simulink model "SPGF_FSK_0000_R2021b"  (R2021b)
settings: Solver=ode4  StartTime=0.0  StopTime=1.4  FixedStep=50e-6/50  RelTol=1e-3  EnableMultiTasking=on
undefined symbols (not defined in the file): D11, Delta
libraries: spsSeriesRLCBranchLib x1645, spsGroundLib x359, spsCurrentMeasurementLib x145, spsIdealSwitchLib x144, spsStairGeneratorLib x135, spsUniversalBridgeLib x76, spsThreePhaseSeriesRLCLoadLib x57, spsSequenceAnalyzerLib x31, simulink x24, spsThreePhaseParallelRLCLoadLib x20, spsThreePhaseTransformerTwoWindingsLib x20, spsDistributedParametersLineLib x19
(part 12 of 36)

== system SPGF_FSK_0000_R2021b/W11/DPL ==
  Ccs2/1 : spsSeriesRLCBranchLib/Series RLC Branch  LConnTagsString=__new0  RConnTagsString=__new0  BranchType=R  Resistance=-Rg_matrix(3,4)*2  Inductance=1e-3  SetiL0=off  InitialCurrent=0  Capacitance=Rg_matrix(3,4)*2  Setx0=off  InitialVoltage=0  Measurements=None
  Ccs2/3 : spsSeriesRLCBranchLib/Series RLC Branch  LConnTagsString=__new0  RConnTagsString=__new0  BranchType=R  Resistance=-Rg_matrix(3,4)*2  Inductance=1e-3  SetiL0=off  InitialCurrent=0  Capacitance=Rg_matrix(3,4)*2  Setx0=off  InitialVoltage=0  Measurements=None
  Ccs3/1 : spsSeriesRLCBranchLib/Series RLC Branch  LConnTagsString=__new0  RConnTagsString=__new0  BranchType=R  Resistance=-Rg_matrix(5,6)*2  Inductance=1e-3  SetiL0=off  InitialCurrent=0  Capacitance=-C_matrix(5,6)/2  Setx0=off  InitialVoltage=0  Measurements=None
  Ccs3/3 : spsSeriesRLCBranchLib/Series RLC Branch  LConnTagsString=__new0  RConnTagsString=__new0  BranchType=R  Resistance=-Rg_matrix(5,6)*2  Inductance=1e-3  SetiL0=off  InitialCurrent=0  Capacitance=-C_matrix(5,6)/2  Setx0=off  InitialVoltage=0  Measurements=None
  DPL : spsDistributedParametersLineLib/Distributed Parameters Line  Phases=6  Length=LineLength  Frequency=Frequency  Resistance=R_matrix  Inductance=L_matrix  Capacitance=C_matrix  x1=[-0.0001055 -1.78412619667985 4844.51130994743 0 0 0 -9280.60987849936;-0.000105 -1.78462942618335 4845.96807552508 0 0 0 -9279.84399978977;-0.0001045 -1.78513261165289 4847.42472153325 0 0 0 -9279.07789210921;-0.000104 -1.78563575307605 4848.88124793602 0 0 0 -9278.31155547658;-0.0001035 -1.78613885044041 4850.33765469743 0 0 0 -9277.54498991079;-0.000103 -1.78664190373356 4851.79394178156 0 0 0 -9276.77819543075;-0.0001025 -1.78714491294309 4853.25010915248 0 0 0 -9276.01117205539;-0.000102 -1.78764787805659 4854.70615677424 0 0 0 -9275.24391980362;-0.0001015 -1.78815079906164 4856.16208461094 0 0 0 -9274.47643869439;-0.000101 -1.78865367594584 4857.61789262663 0 0 0 -9273.70872874662;-0.0001005 -1.78915650869679 4859.07358078542 0 0 0 -9272.94078997926;-0.0001 -1.78965929730206 4860.52914905136 0 0 0 -9272.17262241126;-9.95e-05 -1.79016204174926 4861.98459738856 0 0 0 -9271.40422606157;-9.9e-05 -1.79066474202598 4863.43992576109 0 0 0 -9270.63560094915;-9.85e-05 -1.79116739811982 4864.89513413306 0 0 0 -9269.86674709296;-9.8e-05 -1.79167001001838 4866.35022246855 0 0 0 -9269.09766451198;-9.75e-05 -1.79217257770925 4867.80519073166 0 0 0 -9268.32835322519;-9.7e-05 -1.79267510118004 4869.26003888649 0 0 0 -9267.55881325156;-9.65e-05 -1.79317758041834 4870.71476689715 0 0 0 -9266.78904461008;-9.6e-05 -1.79368001541176 4872.16937472774 0 0 0 -9266.01904731975;-9.55e-05 -1.79418240614789 4873.62386234236 0 0 0 -9265.24882139956;-9.5e-05 -1.79468475261435 4875.07822970514 0 0 0 -9264.47836686852;-9.45e-05 -1.79518705479874 4876.53247678019 0 0 0 -9263.70768374564;-9.4e-05 -1.79568931268867 4877.98660353161 0 0 0 -9262.93677204993;-9.35e-05 -1.79619152627174 4879.44060992355 0 0 0 -9262.16563180043;-9.3e-05 -1.79669369553555 4880.89449592011 0 0 0 -9261.39426301614;-9.25e-05 -1.79719582046773 4882.34826148543 0 0 0 -9260.62266571611;-9.2e-05 -1.79769790105588 4883.80190658364 0 0 0 -9259.85083991938;-9.15e-05 -1.79819993728761 4885.25543117886 0 0 0 -9259.07878564499;-9.1e-05 -1.79870192915053 4886.70883523523 0 0 0 -9258.30650291198;-9.05e-05 -1.79920387663227 4888.1621187169 0 0 0 -9257.53399173942;-9e-05 -1.79970577972043 4889.61528158801 0 0 0 -9256.76125214637;-8.95e-05 -1.80020763840262 4891.06832381269 0 0 0 -9255.98828415188;-8.9e-05 -1.80070945266648 4892.5212453551 0 0 0 -9255.21508777504;-8.85e-05 -1.80121122249961 4893.97404617938 0 0 0 -9254.44166303492;-8.8e-05 -1.80171294788964 4895.4267262497 0 0 0 -9253.6680099506;-8.75e-05 -1.80221462882418 4896.87928553021 0 0 0 -9252.89412854118;-8.7e-05 -1.80271626529085 4898.33172398506 0 0 0 -9252.12001882575;-8.65e-05 -1.80321785727729 4899.78404157842 0 0 0 -9251.34568082341;-8.6e-05 -1.80371940477111 4901.23623827445 0 0 0 -9250.57111455326;-8.55e-05 -1.80422090775993 4902.68831403733 0 0 0 -9249.79632003442;-8.5e-05 -1.80472236623139 4904.14026883123 0 0 0 -9249.02129728601;-8.45e-05 -1.80522378017311 4905.59210262031 0 0 0 -9248.24604632714;-8.4e-05 -1.80572514957272 4907.04381536876 0 0 0 -9247.47056717695;-8.35e-05 -1.80622647441785 4908.49540704076 0 0 0 -9246.69485985456;-8.3e-05 -1.80672775469612 4909.94687760048 0 0 0 -9245.91892437913;-8.25e-05 -1.80722899039518 4911.39822701213 0 0 0 -9245.14276076979;-8.2e-05 -1.80773018150264 4912.84945523988 0 0 0 -9244.3663690457;-8.15e-05 -1.80823132800616 4914.30056224793 0 0 0 -9243.58974922601;-8.1e-05 -1.80873242989335 4915.75154800047 0 0 0 -9242.81290132989;-8.05e-05 -1.80923348715186 4917.20241246171 0 0 0 -9242.0358253765;-8e-05 -1.80973449976932 4918.65315559584 0 0 0 -9241.25852138502;-7.95e-05 -1.81023546773337 4920.10377736707 0 0 0 -9240.48098937462;-7.9e-05 -1.81073639103166 4921.5542777396 0 0 0 -9239.70322936449;-7.85e-05 -1.81123726965181 4923.00465667765 0 0 0 -9238.92524137383;-7.8e-05 -1.81173810358148 4924.45491414543 0 0 0 -9238.14702542182;-7.75e-05 -1.8122388928083 4925.90505010715 0 0 0 -9237.36858152767;-7.7e-05 -1.81273963731991 4927.35506452704 0 0 0 -9236.58990971059;-7.65e-05 -1.81324033710397 ...(+12181 chars)]  x2=[-0.0001055 -1.77906835575681 4945.74076916884 0 0 0 -9459.89906055918;-0.000105 -1.7795989916804 4947.22756988038 0 0 0 -9459.12257831348;-0.0001045 -1.78012958369414 4948.71424852397 0 0 0 -9458.34586267329;-0.000104 -1.78066013178495 4950.20080506292 0 0 0 -9457.56891365777;-0.0001035 -1.78119063593973 4951.68723946057 0 0 0 -9456.79173128609;-0.000103 -1.78172109614539 4953.17355168024 0 0 0 -9456.01431557743;-0.0001025 -1.78225151238884 4954.65974168524 0 0 0 -9455.23666655097;-0.000102 -1.782781884657 4956.14580943892 0 0 0 -9454.4587842259;-0.0001015 -1.78331221293679 4957.6317549046 0 0 0 -9453.68066862141;-0.000101 -1.7838424972151 4959.11757804562 0 0 0 -9452.90231975669;-0.0001005 -1.78437273747887 4960.60327882532 0 0 0 -9452.12373765096;-0.0001 -1.78490293371501 4962.08885720704 0 0 0 -9451.34492232343;-9.95e-05 -1.78543308591043 4963.57431315412 0 0 0 -9450.56587379331;-9.9e-05 -1.78596319405205 4965.05964662992 0 0 0 -9449.78659207982;-9.85e-05 -1.7864932581268 4966.54485759778 0 0 0 -9449.00707720219;-9.8e-05 -1.7870232781216 4968.02994602106 0 0 0 -9448.22732917966;-9.75e-05 -1.78755325402336 4969.51491186311 0 0 0 -9447.44734803147;-9.7e-05 -1.78808318581901 4970.9997550873 0 0 0 -9446.66713377685;-9.65e-05 -1.78861307349548 4972.48447565699 0 0 0 -9445.88668643507;-9.6e-05 -1.7891429170397 4973.96907353554 0 0 0 -9445.10600602538;-9.55e-05 -1.78967271643858 4975.45354868632 0 0 0 -9444.32509256703;-9.5e-05 -1.79020247167905 4976.93790107271 0 0 0 -9443.54394607931;-9.45e-05 -1.79073218274805 4978.42213065807 0 0 0 -9442.76256658148;-9.4e-05 -1.79126184963251 4979.9062374058 0 0 0 -9441.98095409282;-9.35e-05 -1.79179147231935 4981.39022127926 0 0 0 -9441.19910863263;-9.3e-05 -1.79232105079551 4982.87408224185 0 0 0 -9440.41703022018;-9.25e-05 -1.79285058504792 4984.35782025695 0 0 0 -9439.63471887477;-9.2e-05 -1.79338007506351 4985.84143528794 0 0 0 -9438.85217461572;-9.15e-05 -1.79390952082923 4987.32492729823 0 0 0 -9438.06939746233;-9.1e-05 -1.794438922332 4988.80829625122 0 0 0 -9437.28638743391;-9.05e-05 -1.79496827955876 4990.29154211029 0 0 0 -9436.50314454978;-9e-05 -1.79549759249646 4991.77466483885 0 0 0 -9435.71966882926;-8.95e-05 -1.79602686113203 4993.25766440031 0 0 0 -9434.9359602917;-8.9e-05 -1.79655608545242 4994.74054075808 0 0 0 -9434.15201895643;-8.85e-05 -1.79708526544456 4996.22329387556 0 0 0 -9433.36784484278;-8.8e-05 -1.7976144010954 4997.70592371617 0 0 0 -9432.58343797011;-8.75e-05 -1.79814349239188 4999.18843024334 0 0 0 -9431.79879835778;-8.7e-05 -1.79867253932095 5000.67081342047 0 0 0 -9431.01392602514;-8.65e-05 -1.79920154186955 5002.153073211 0 0 0 -9430.22882099156;-8.6e-05 -1.79973050002464 5003.63520957835 0 0 0 -9429.4434832764;-8.55e-05 -1.80025941377315 5005.11722248594 0 0 0 -9428.65791289906;-8.5e-05 -1.80078828310204 5006.59911189723 0 0 0 -9427.87210987891;-8.45e-05 -1.80131710799827 5008.08087777562 0 0 0 -9427.08607423534;-8.4e-05 -1.80184588844877 5009.56252008458 0 0 0 -9426.29980598774;-8.35e-05 -1.80237462444052 5011.04403878754 0 0 0 -9425.51330515552;-8.3e-05 -1.80290331596045 5012.52543384794 0 0 0 -9424.72657175808;-8.25e-05 -1.80343196299552 5014.00670522923 0 0 0 -9423.93960581483;-8.2e-05 -1.80396056553269 5015.48785289487 0 0 0 -9423.1524073452;-8.15e-05 -1.80448912355892 5016.9688768083 0 0 0 -9422.3649763686;-8.1e-05 -1.80501763706117 5018.44977693299 0 0 0 -9421.57731290446;-8.05e-05 -1.80554610602639 5019.9305532324 0 0 0 -9420.78941697222;-8e-05 -1.80607453044155 5021.41120566998 0 0 0 -9420.00128859132;-7.95e-05 -1.8066029102936 5022.89173420921 0 0 0 -9419.21292778121;-7.9e-05 -1.80713124556952 5024.37213881355 0 0 0 -9418.42433456133;-7.85e-05 -1.80765953625626 5025.85241944648 0 0 0 -9417.63550895114;-7.8e-05 -1.80818778234078 5027.33257607148 0 0 0 -9416.84645097012;-7.75e-05 -1.80871598381007 5028.81260865201 0 0 0 -9416.05716063772;-7.7e-05 -1.80924414065107 5030.29251715156 0 0 0 -9415.26763797342;-7.65e-05 -1.80977225285076 ...(+12156 chars)]  x3=[-0.0001055 0.0207090066909794 -36.7832656385474 0 0 0 -561.751834737637;-0.000105 0.0207044314271113 -36.6997989422163 0 0 0 -561.75382588602;-0.0001045 0.0206998556523819 -36.616331340354 0 0 0 -561.755803173683;-0.000104 0.0206952793669039 -36.5328628350199 0 0 0 -561.757766600577;-0.0001035 0.0206907025707905 -36.4493934282735 0 0 0 -561.759716166653;-0.000103 0.0206861252641544 -36.3659231221744 0 0 0 -561.761651871865;-0.0001025 0.0206815474471086 -36.2824519187821 0 0 0 -561.763573716163;-0.000102 0.0206769691197661 -36.1989798201562 0 0 0 -561.7654816995;-0.0001015 0.0206723902822399 -36.1155068283563 0 0 0 -561.76737582183;-0.000101 0.0206678109346428 -36.0320329454419 0 0 0 -561.769256083106;-0.0001005 0.020663231077088 -35.9485581734728 0 0 0 -561.771122483281;-0.0001 0.0206586507096883 -35.8650825145086 0 0 0 -561.772975022309;-9.95e-05 0.0206540698325569 -35.7816059706089 0 0 0 -561.774813700144;-9.9e-05 0.0206494884458068 -35.6981285438335 0 0 0 -561.776638516741;-9.85e-05 0.0206449065495509 -35.614650236242 0 0 0 -561.778449472056;-9.8e-05 0.0206403241439024 -35.5311710498943 0 0 0 -561.780246566043;-9.75e-05 0.0206357412289744 -35.4476909868501 0 0 0 -561.782029798658;-9.7e-05 0.0206311578048798 -35.3642100491692 0 0 0 -561.783799169857;-9.65e-05 0.0206265738717318 -35.2807282389114 0 0 0 -561.785554679596;-9.6e-05 0.0206219894296434 -35.1972455581365 0 0 0 -561.787296327833;-9.55e-05 0.0206174044787279 -35.1137620089044 0 0 0 -561.789024114524;-9.5e-05 0.0206128190190984 -35.0302775932749 0 0 0 -561.790738039626;-9.45e-05 0.0206082330508679 -34.946792313308 0 0 0 -561.792438103097;-9.4e-05 0.0206036465741496 -34.8633061710635 0 0 0 -561.794124304895;-9.35e-05 0.0205990595890567 -34.7798191686015 0 0 0 -561.795796644979;-9.3e-05 0.0205944720957025 -34.6963313079818 0 0 0 -561.797455123308;-9.25e-05 0.0205898840941999 -34.6128425912644 0 0 0 -561.79909973984;-9.2e-05 0.0205852955846624 -34.5293530205094 0 0 0 -561.800730494535;-9.15e-05 0.0205807065672031 -34.4458625977768 0 0 0 -561.802347387352;-9.1e-05 0.0205761170419351 -34.3623713251266 0 0 0 -561.803950418252;-9.05e-05 0.0205715270089719 -34.2788792046188 0 0 0 -561.805539587195;-9e-05 0.0205669364684265 -34.1953862383136 0 0 0 -561.807114894143;-8.95e-05 0.0205623454204124 -34.111892428271 0 0 0 -561.808676339055;-8.9e-05 0.0205577538650427 -34.0283977765513 0 0 0 -561.810223921894;-8.85e-05 0.0205531618024307 -33.9449022852145 0 0 0 -561.811757642621;-8.8e-05 0.0205485692326898 -33.8614059563208 0 0 0 -561.813277501199;-8.75e-05 0.0205439761559333 -33.7779087919304 0 0 0 -561.81478349759;-8.7e-05 0.0205393825722745 -33.6944107941035 0 0 0 -561.816275631757;-8.65e-05 0.0205347884818268 -33.6109119649004 0 0 0 -561.817753903662;-8.6e-05 0.0205301938847034 -33.5274123063812 0 0 0 -561.819218313271;-8.55e-05 0.0205255987810179 -33.4439118206063 0 0 0 -561.820668860546;-8.5e-05 0.0205210031708834 -33.360410509636 0 0 0 -561.822105545451;-8.45e-05 0.0205164070544135 -33.2769083755305 0 0 0 -561.823528367952;-8.4e-05 0.0205118104317216 -33.1934054203502 0 0 0 -561.824937328013;-8.35e-05 0.020507213302921 -33.1099016461555 0 0 0 -561.826332425599;-8.3e-05 0.0205026156681253 -33.0263970550067 0 0 0 -561.827713660676;-8.25e-05 0.0204980175274477 -32.9428916489642 0 0 0 -561.82908103321;-8.2e-05 0.0204934188810019 -32.8593854300884 0 0 0 -561.830434543167;-8.15e-05 0.0204888197289012 -32.7758784004398 0 0 0 -561.831774190514;-8.1e-05 0.0204842200712592 -32.6923705620789 0 0 0 -561.833099975217;-8.05e-05 0.0204796199081892 -32.608861917066 0 0 0 -561.834411897245;-8e-05 0.0204750192398049 -32.5253524674617 0 0 0 -561.835709956563;-7.95e-05 0.0204704180662198 -32.4418422153265 0 0 0 -561.836994153142;-7.9e-05 0.0204658163875474 -32.3583311627209 0 0 0 -561.838264486948;-7.85e-05 0.0204612142039011 -32.2748193117055 0 0 0 -561.839520957951;-7.8e-05 0.0204566115153947 -32.1913066643409 0 0 0 -561.840763566119;-7.75e-05 0.0204520083221416 -32.1077932226876 0 0 0 ...(+12583 chars)]  x4=[-0.0001055 -0.04304225965487 184.459272299607 0 0 0 227.528775566243;-0.000105 -0.0430444284629222 184.420510607988 0 0 0 227.558114219598;-0.0001045 -0.0430465962088957 184.381744365975 0 0 0 227.587447258182;-0.000104 -0.043048762892737 184.342973574525 0 0 0 227.61677468127;-0.0001035 -0.0430509285143927 184.304198234594 0 0 0 227.64609648814;-0.000103 -0.0430530930738093 184.26541834714 0 0 0 227.675412678067;-0.0001025 -0.0430552565709334 184.226633913118 0 0 0 227.704723250329;-0.000102 -0.0430574190057116 184.187844933487 0 0 0 227.734028204201;-0.0001015 -0.0430595803780906 184.149051409203 0 0 0 227.763327538962;-0.000101 -0.043061740688017 184.110253341223 0 0 0 227.792621253888;-0.0001005 -0.0430638999354376 184.071450730505 0 0 0 227.821909348257;-0.0001 -0.0430660581202991 184.032643578005 0 0 0 227.851191821345;-9.95e-05 -0.0430682152425481 183.993831884682 0 0 0 227.88046867243;-9.9e-05 -0.0430703713021315 183.955015651494 0 0 0 227.90973990079;-9.85e-05 -0.0430725262989961 183.916194879397 0 0 0 227.939005505703;-9.8e-05 -0.0430746802330888 183.87736956935 0 0 0 227.968265486446;-9.75e-05 -0.0430768331043563 183.838539722311 0 0 0 227.997519842298;-9.7e-05 -0.0430789849127455 183.799705339238 0 0 0 228.026768572537;-9.65e-05 -0.0430811356582034 183.760866421089 0 0 0 228.05601167644;-9.6e-05 -0.0430832853406769 183.722022968822 0 0 0 228.085249153287;-9.55e-05 -0.043085433960113 183.683174983396 0 0 0 228.114481002356;-9.5e-05 -0.0430875815164585 183.644322465769 0 0 0 228.143707222926;-9.45e-05 -0.0430897280096606 183.6054654169 0 0 0 228.172927814275;-9.4e-05 -0.0430918734396663 183.566603837748 0 0 0 228.202142775683;-9.35e-05 -0.0430940178064227 183.527737729272 0 0 0 228.231352106429;-9.3e-05 -0.0430961611098767 183.48886709243 0 0 0 228.260555805792;-9.25e-05 -0.0430983033499756 183.449991928182 0 0 0 228.289753873052;-9.2e-05 -0.0431004445266665 183.411112237487 0 0 0 228.318946307488;-9.15e-05 -0.0431025846398966 183.372228021304 0 0 0 228.348133108379;-9.1e-05 -0.043104723689613 183.333339280593 0 0 0 228.377314275007;-9.05e-05 -0.043106861675763 183.294446016312 0 0 0 228.40648980665;-9e-05 -0.0431089985982938 183.255548229423 0 0 0 228.435659702588;-8.95e-05 -0.0431111344571527 183.216645920884 0 0 0 228.464823962103;-8.9e-05 -0.0431132692522871 183.177739091656 0 0 0 228.493982584474;-8.85e-05 -0.0431154029836441 183.138827742698 0 0 0 228.523135568982;-8.8e-05 -0.0431175356511712 183.099911874971 0 0 0 228.552282914908;-8.75e-05 -0.0431196672548157 183.060991489434 0 0 0 228.581424621532;-8.7e-05 -0.0431217977945252 183.022066587049 0 0 0 228.610560688136;-8.65e-05 -0.0431239272702469 182.983137168775 0 0 0 228.639691114;-8.6e-05 -0.0431260556819283 182.944203235573 0 0 0 228.668815898406;-8.55e-05 -0.043128183029517 182.905264788404 0 0 0 228.697935040635;-8.5e-05 -0.0431303093129604 182.866321828228 0 0 0 228.727048539968;-8.45e-05 -0.0431324345322061 182.827374356007 0 0 0 228.756156395688;-8.4e-05 -0.0431345586872017 182.788422372701 0 0 0 228.785258607076;-8.35e-05 -0.0431366817778946 182.749465879272 0 0 0 228.814355173415;-8.3e-05 -0.0431388038042326 182.71050487668 0 0 0 228.843446093985;-8.25e-05 -0.0431409247661633 182.671539365887 0 0 0 228.872531368069;-8.2e-05 -0.0431430446636343 182.632569347855 0 0 0 228.90161099495;-8.15e-05 -0.0431451634965934 182.593594823545 0 0 0 228.930684973911;-8.1e-05 -0.0431472812649883 182.554615793918 0 0 0 228.959753304233;-8.05e-05 -0.0431493979687666 182.515632259937 0 0 0 228.988815985199;-8e-05 -0.0431515136078763 182.476644222563 0 0 0 229.017873016093;-7.95e-05 -0.043153628182265 182.437651682758 0 0 0 229.046924396198;-7.9e-05 -0.0431557416918806 182.398654641485 0 0 0 229.075970124796;-7.85e-05 -0.043157854136671 182.359653099705 0 0 0 229.105010201171;-7.8e-05 -0.043159965516584 182.320647058381 0 0 0 229.134044624607;-7.75e-05 -0.0431620758315675 182.281636518476 0 0 0 229.163073394387;-7.7e-05 -0.0431641850815695 182.242621480951 0 0 0 ...(+12359 chars)]  x5=0.000105022628283662  V1=ones(3,3)  V2=ones(3,3)  I1=ones(3,3)  I2=ones(3,3)  nHarmo=1  Measurements=None  Decoupling=off  VsMag0=0  VrMag0=0  VsAngle0=0  VrAngle0=0  IsMag0=0  IrMag0=0  IsAngle0=0  IrAngle0=0
  Ground{1..4} (4 alike) : spsGroundLib/Ground  LConnTagsString=a
  Rcs*1 : spsSeriesRLCBranchLib/Series RLC Branch  LConnTagsString=__new0  RConnTagsString=__new0  BranchType=R  Resistance=-Rg_matrix(1,2)*2  Inductance=1e-3  SetiL0=off  InitialCurrent=0  Capacitance=Rg_matrix(1,2)*2  Setx0=off  InitialVoltage=0  Measurements=None
  Rcs*2 : spsSeriesRLCBranchLib/Series RLC Branch  LConnTagsString=__new0  RConnTagsString=__new0  BranchType=R  Resistance=-Rg_matrix(1,2)*2  Inductance=1e-3  SetiL0=off  InitialCurrent=0  Capacitance=Rg_matrix(1,2)*2  Setx0=off  InitialVoltage=0  Measurements=None
  Rgsg1/1 : spsSeriesRLCBranchLib/Series RLC Branch  LConnTagsString=__new0  RConnTagsString=__new0  BranchType=R  Resistance=(Rg_matrix(4,4)+Rg_matrix(3,4))*2  Inductance=1e-3  SetiL0=off  InitialCurrent=0  Capacitance=Rg_matrix(1,2)*2  Setx0=off  InitialVoltage=0  Measurements=None
  Rgsg1/2 : spsSeriesRLCBranchLib/Series RLC Branch  LConnTagsString=__new0  RConnTagsString=__new0  BranchType=R  Resistance=(Rg_matrix(2,2)+Rg_matrix(1,2))*2  Inductance=1e-3  SetiL0=off  InitialCurrent=0  Capacitance=Rg_matrix(1,2)*2  Setx0=off  InitialVoltage=0  Measurements=None
  Rgsg1/3 : spsSeriesRLCBranchLib/Series RLC Branch  LConnTagsString=__new0  RConnTagsString=__new0  BranchType=R  Resistance=(Rg_matrix(4,4)+Rg_matrix(3,4))*2  Inductance=1e-3  SetiL0=off  InitialCurrent=0  Capacitance=Rg_matrix(1,2)*2  Setx0=off  InitialVoltage=0  Measurements=None
  Rgsg1/4 : spsSeriesRLCBranchLib/Series RLC Branch  LConnTagsString=__new0  RConnTagsString=__new0  BranchType=R  Resistance=(Rg_matrix(2,2)+Rg_matrix(1,2))*2  Inductance=1e-3  SetiL0=off  InitialCurrent=0  Capacitance=Rg_matrix(1,2)*2  Setx0=off  InitialVoltage=0  Measurements=None
  Rsg*1 : spsSeriesRLCBranchLib/Series RLC Branch  LConnTagsString=__new0  RConnTagsString=__new0  BranchType=R  Resistance=(Rg_matrix(6,6)+Rg_matrix(5,6))*2  Inductance=1e-3  SetiL0=off  InitialCurrent=0  Capacitance=Rg_matrix(1,2)*2  Setx0=off  InitialVoltage=0  Measurements=None
  Rsg*2 : spsSeriesRLCBranchLib/Series RLC Branch  LConnTagsString=__new0  RConnTagsString=__new0  BranchType=R  Resistance=(Rg_matrix(6,6)+Rg_matrix(5,6))*2  Inductance=1e-3  SetiL0=off  InitialCurrent=0  Capacitance=Rg_matrix(1,2)*2  Setx0=off  InitialVoltage=0  Measurements=None
  A : PMIOPort  Side=Left
  B : PMIOPort  Port=2  Side=Left
  C : PMIOPort  Port=3  Side=Left
  a : PMIOPort  Port=4  Side=Right
  b : PMIOPort  Port=5  Side=Right
  c : PMIOPort  Port=6  Side=Right
  connections:
  DPL/LConn2 -- Rgsg1/1/LConn1 -- Ccs2/3/LConn1 -- DPL/LConn4 -- Ccs3/3/LConn1 -- Rsg*2/LConn1 -- DPL/LConn6 -- Ground3/LConn1 -- Rgsg1/2/LConn1 -- Rcs*2/LConn1
  DPL/RConn5 -- c/RConn1 -- Ccs3/1/RConn1
  Ccs2/1/RConn1 -- b/RConn1 -- DPL/RConn3
  DPL/RConn1 -- a/RConn1 -- Rcs*1/RConn1
  DPL/RConn6 -- Ground4/LConn1 -- Rgsg1/4/LConn1 -- Rcs*1/LConn1 -- DPL/RConn2 -- Rgsg1/3/LConn1 -- Ccs2/1/LConn1 -- DPL/RConn4 -- Ccs3/1/LConn1 -- Rsg*1/LConn1
  Rgsg1/3/RConn1 -- Ground1/LConn1 -- Rgsg1/4/RConn1 -- Rsg*1/RConn1
  Rgsg1/2/RConn1 -- Ground2/LConn1 -- Rgsg1/1/RConn1 -- Rsg*2/RConn1
  DPL/LConn5 -- Ccs3/3/RConn1 -- C/RConn1
  DPL/LConn3 -- Ccs2/3/RConn1 -- B/RConn1
  DPL/LConn1 -- Rcs*2/RConn1 -- A/RConn1
